simulink model "liftTests_2015b"  (R2015b)
settings: Solver=VariableStepAuto  SolverMode=SingleTasking  StartTime=0.0  StopTime=10.0  RelTol=1e-3
undefined symbols (not defined in the file or in its folder): sigbuilder_block
settings Model: Creator=User  LastModifiedBy=User
settings DataIOCC: LimitDataPoints=off  ReturnWorkspaceOutputs=on
settings DebuggingCC: AllowSymbolicDim=on  SFUnexpectedBacktrackingDiag=error  SFNoUnconditionalDefaultTransitionDiag=error
settings ModelReferenceCC: PropagateSignalLabelsOutOfModel=on
settings SFSimCC: SimUseLocalCustomCode=on
settings RTWCC: RTWUseLocalCustomCode=on
settings GRTTargetCC: TargetLangStandard=C99 (ISO)
settings ConfigComp: CovMetricSettings=dwe  CovHtmlReporting=off  CovSaveCumulativeToWorkspaceVar=off  CovSaveSingleToWorkspaceVar=off  CovModelRefEnable=Off  CovExternalEMLEnable=on

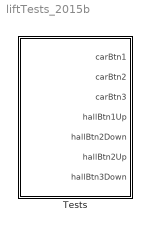
== system liftTests_2015b ==
  Tests : Subsystem  Tag=STV Subsys  LoadFcn=sigbuilder_block('load');  StartFcn=sigbuilder_block('start');  StopFcn=sigbuilder_block('stop');  ClipboardFcn=sigbuilder_block('clipboard');  mask(Sigbuilder block){}
      mask help: Simulink:masks:SigbuilderBlock_MD
      mask init:
      | if ~strcmp(get_param(bdroot(gcbh),'SimulationStatus'),'stopped') tuvar = sigbuilder_block('maskInit'); end
      settings: CopyFcn=sigbuilder_block('copy');  DeleteFcn=sigbuilder_block('delete');  ModelCloseFcn=sigbuilder_block('modelClose');  PreSaveFcn=sigbuilder_block('preSave');  PauseFcn=sigbuilder_block('pause');  ContinueFcn=sigbuilder_block('continue');  NameChangeFcn=sigbuilder_block('namechange');  OpenFcn=sigbuilder_block('open',[9.6 82.8 575.4 499.8 ]);  CloseFcn=sigbuilder_block('close');
      mask Display: plot(0, 0, 100, 100,[2, 2, 32, 32, 2], [68, 8, 8, 68, 68],[32, 2], [38, 38], [32, 19, 2],[53, 60, 44], [32, 17, 17, 2],[16, 16, 31, 31]);txt = getActiveGroup(gcbh);text(2, 100, txt,'verticalAlignment', 'top');

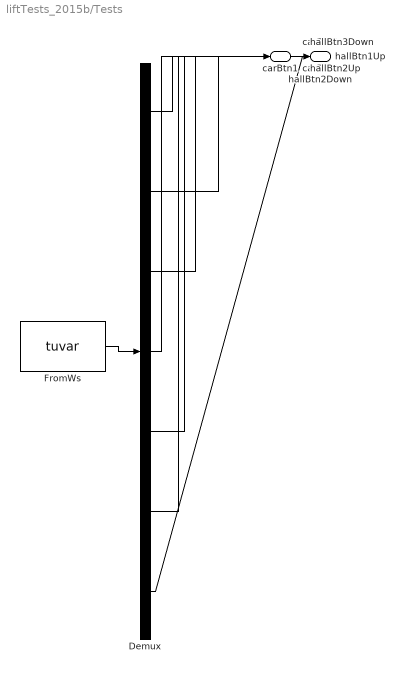
== system liftTests_2015b/Tests ==
  Demux : Demux  Tag=STV Demux  Outputs=7
      settings: DisplayOption=none
  FromWs : FromWorkspace  Tag=STV FromWs  VariableName=tuvar
      SigBuilderData=|
      | common.afterFinalStr = 'Extrapolate'
      | common.sampleTime = 0
      | dataSet(1).timeRange = [0 40]
      | dataSet(1).name = 'carBtns test'
      | dataSet(2).timeRange = [0 40]
      | dataSet(2).name = 'hallBtns test'
      | dataSet(3).timeRange = [0 40]
      | dataSet(3).name = 'queue test - Scenario1 - insert in the middle'
      | dataSet(4).timeRange = [0 40]
      | dataSet(4).name = 'queue test - Scenario1 - insert at the end'
      | dataSet(5).timeRange = [0 40]
      | dataSet(5).name = 'queue test - Scenario2 - inset at the end'
      | sbobj.Groups(1).Name = 'carBtns test'
      | sbobj.Groups(1).Signals(1).Name = 'carBtn1'
      | sbobj.Groups(1).Signals(1).XData = [0 13 13 14 14 40]
      | sbobj.Groups(1).Signals(1).YData = [0 0 1 1 0 0]
      | sbobj.Groups(1).Signals(2).Name = 'carBtn2'
      | sbobj.Groups(1).Signals(2).XData = [0 3 3 4 4 40]
      | sbobj.Groups(1).Signals(2).YData = [0 0 1 1 0 0]
      | sbobj.Groups(1).Signals(3).Name = 'carBtn3'
      | sbobj.Groups(1).Signals(3).XData = [0 8 8 9 9 40]
      | sbobj.Groups(1).Signals(3).YData = [0 0 1 1 0 0]
      | sbobj.Groups(1).Signals(4).Name = 'hallBtn1Up'
      | sbobj.Groups(1).Signals(4).XData = [0 16 24 40]
      | sbobj.Groups(1).Signals(4).YData = [0 0 0 0]
      | sbobj.Groups(1).Signals(5).Name = 'hallBtn2Down'
      | sbobj.Groups(1).Signals(5).XData = [0 16 24 40]
      | sbobj.Groups(1).Signals(5).YData = [0 0 0 0]
      | sbobj.Groups(1).Signals(6).Name = 'hallBtn2Up'
      | sbobj.Groups(1).Signals(6).XData = [0 16 24 40]
      | sbobj.Groups(1).Signals(6).YData = [0 0 0 0]
      | sbobj.Groups(1).Signals(7).Name = 'hallBtn3Down'
      | sbobj.Groups(1).Signals(7).XData = [0 16 24 40]
      | sbobj.Groups(1).Signals(7).YData = [0 0 0 0]
      | sbobj.Groups(1).TimeRange = [0 40]
      | sbobj.Groups(2).Name = 'hallBtns test'
      | sbobj.Groups(2).Signals(1).Name = 'carBtn1'
      | sbobj.Groups(2).Signals(1).XData = [0 13 14 40]
      | sbobj.Groups(2).Signals(1).YData = [0 0 0 0]
      | sbobj.Groups(2).Signals(2).Name = 'carBtn2'
      | sbobj.Groups(2).Signals(2).XData = [0 3 4 40]
      | sbobj.Groups(2).Signals(2).YData = [0 0 0 0]
      | sbobj.Groups(2).Signals(3).Name = 'carBtn3'
      | sbobj.Groups(2).Signals(3).XData = [0 8 9 40]
      | sbobj.Groups(2).Signals(3).YData = [0 0 0 0]
      | sbobj.Groups(2).Signals(4).Name = 'hallBtn1Up'
      | sbobj.Groups(2).Signals(4).XData = [0 20 20 21 21 40]
      | sbobj.Groups(2).Signals(4).YData = [0 0 1 1 0 0]
      | sbobj.Groups(2).Signals(5).Name = 'hallBtn2Down'
      | sbobj.Groups(2).Signals(5).XData = [0 25 25 26 26 40]
      | sbobj.Groups(2).Signals(5).YData = [0 0 1 1 0 0]
      | sbobj.Groups(2).Signals(6).Name = 'hallBtn2Up'
      | sbobj.Groups(2).Signals(6).XData = [0 5 5 6 6 40]
      | sbobj.Groups(2).Signals(6).YData = [0 0 1 1 0 0]
      | sbobj.Groups(2).Signals(7).Name = 'hallBtn3Down'
      | sbobj.Groups(2).Signals(7).XData = [0 10 10 11 11 40]
      | sbobj.Groups(2).Signals(7).YData = [0 0 1 1 0 0]
      | sbobj.Groups(2).TimeRange = [0 40]
      | sbobj.Groups(3).Name = 'queue test - Scenario1 - insert in the middle'
      | sbobj.Groups(3).Signals(1).Name = 'carBtn1'
      | sbobj.Groups(3).Signals(1).XData = [0 13 14 40]
      | sbobj.Groups(3).Signals(1).YData = [0 0 0 0]
      | sbobj.Groups(3).Signals(2).Name = 'carBtn2'
      | sbobj.Groups(3).Signals(2).XData = [0 7 7 8 8 40]
      | sbobj.Groups(3).Signals(2).YData = [0 0 1 1 0 0]
      | sbobj.Groups(3).Signals(3).Name = 'carBtn3'
      | sbobj.Groups(3).Signals(3).XData = [0 8 9 40]
      | sbobj.Groups(3).Signals(3).YData = [0 0 0 0]
      | sbobj.Groups(3).Signals(4).Name = 'hallBtn1Up'
      | sbobj.Groups(3).Signals(4).XData = [0 20 21 40]
      | sbobj.Groups(3).Signals(4).YData = [0 0 0 0]
      | sbobj.Groups(3).Signals(5).Name = 'hallBtn2Down'
      | sbobj.Groups(3).Signals(5).XData = [0 25 26 40]
      | sbobj.Groups(3).Signals(5).YData = [0 0 0 0]
      | sbobj.Groups(3).Signals(6).Name = 'hallBtn2Up'
      | sbobj.Groups(3).Signals(6).XData = [0 5 6 40]
      | sbobj.Groups(3).Signals(6).YData = [0 0 0 0]
      | sbobj.Groups(3).Signals(7).Name = 'hallBtn3Down'
      | sbobj.Groups(3).Signals(7).XData = [0 5 5 6 6 40]
      | sbobj.Groups(3).Signals(7).YData = [0 0 1 1 0 0]
      | sbobj.Groups(3).TimeRange = [0 40]
      | sbobj.Groups(4).Name = 'queue test - Scenario1 - insert at the end'
      | sbobj.Groups(4).Signals(1).Name = 'carBtn1'
      | sbobj.Groups(4).Signals(1).XData = [0 13 14 40]
      | sbobj.Groups(4).Signals(1).YData = [0 0 0 0]
      | sbobj.Groups(4).Signals(2).Name = 'carBtn2'
      | sbobj.Groups(4).Signals(2).XData = [0 11 11 12 12 40]
      | sbobj.Groups(4).Signals(2).YData = [0 0 1 1 0 0]
      | sbobj.Groups(4).Signals(3).Name = 'carBtn3'
      | sbobj.Groups(4).Signals(3).XData = [0 8 9 40]
      | sbobj.Groups(4).Signals(3).YData = [0 0 0 0]
      | sbobj.Groups(4).Signals(4).Name = 'hallBtn1Up'
      | sbobj.Groups(4).Signals(4).XData = [0 20 21 40]
      | sbobj.Groups(4).Signals(4).YData = [0 0 0 0]
      | sbobj.Groups(4).Signals(5).Name = 'hallBtn2Down'
      | sbobj.Groups(4).Signals(5).XData = [0 25 26 40]
      | sbobj.Groups(4).Signals(5).YData = [0 0 0 0]
      | sbobj.Groups(4).Signals(6).Name = 'hallBtn2Up'
      | sbobj.Groups(4).Signals(6).XData = [0 5 6 40]
      | sbobj.Groups(4).Signals(6).YData = [0 0 0 0]
      | sbobj.Groups(4).Signals(7).Name = 'hallBtn3Down'
      | sbobj.Groups(4).Signals(7).XData = [0 5 5 6 6 40]
      | sbobj.Groups(4).Signals(7).YData = [0 0 1 1 0 0]
      | sbobj.Groups(4).TimeRange = [0 40]
      | sbobj.Groups(5).Name = 'queue test - Scenario2 - inset at the end'
      | sbobj.Groups(5).Signals(1).Name = 'carBtn1'
      | sbobj.Groups(5).Signals(1).XData = [0 13 14 40]
      | sbobj.Groups(5).Signals(1).YData = [0 0 0 0]
      | sbobj.Groups(5).Signals(2).Name = 'carBtn2'
      | sbobj.Groups(5).Signals(2).XData = [0 6 7 40]
      | sbobj.Groups(5).Signals(2).YData = [0 0 0 0]
      | sbobj.Groups(5).Signals(3).Name = 'carBtn3'
      | sbobj.Groups(5).Signals(3).XData = [0 5 5 6 6 40]
      | sbobj.Groups(5).Signals(3).YData = [0 0 1 1 0 0]
      | sbobj.Groups(5).Signals(4).Name = 'hallBtn1Up'
      | sbobj.Groups(5).Signals(4).XData = [0 20 21 40]
      | sbobj.Groups(5).Signals(4).YData = [0 0 0 0]
      | sbobj.Groups(5).Signals(5).Name = 'hallBtn2Down'
      | sbobj.Groups(5).Signals(5).XData = [0 6.5 6.5 7.5 7.5 40]
      | sbobj.Groups(5).Signals(5).YData = [0 0 1 1 0 0]
      | sbobj.Groups(5).Signals(6).Name = 'hallBtn2Up'
      | sbobj.Groups(5).Signals(6).XData = [0 5 6 40]
      | sbobj.Groups(5).Signals(6).YData = [0 0 0 0]
      | sbobj.Groups(5).Signals(7).Name = 'hallBtn3Down'
      | sbobj.Groups(5).Signals(7).XData = [0 5 6 40]
      | sbobj.Groups(5).Signals(7).YData = [0 0 0 0]
      | sbobj.Groups(5).TimeRange = [0 40]
  carBtn1 : Outport  Tag=STV Outport
  carBtn2 : Outport  Tag=STV Outport  Port=2
  carBtn3 : Outport  Tag=STV Outport  Port=3
  hallBtn1Up : Outport  Tag=STV Outport  Port=4
  hallBtn2Down : Outport  Tag=STV Outport  Port=5
  hallBtn2Up : Outport  Tag=STV Outport  Port=6
  hallBtn3Down : Outport  Tag=STV Outport  Port=7
  wires:
  Demux/1 -> carBtn1/1
  FromWs/1 -> Demux/1
  Demux/2 -> carBtn2/1
  Demux/3 -> carBtn3/1
  Demux/4 -> hallBtn1Up/1
  Demux/5 -> hallBtn2Down/1
  Demux/6 -> hallBtn2Up/1
  Demux/7 -> hallBtn3Down/1
